simulink model "PID_Tavola1"  (R2018b)
settings: Solver=FixedStepAuto  StartTime=0.0  StopTime=10  FixedStep=0.1  RelTol=1e-3
values from neighbouring files (symbols this model uses):
  cond_init = [x1,x2,x3,x4,x5,x6]'    [main.m]
  Law = [10,4,4,4,4,4 ... (first row only)    [main.m]
  param = param'    [main.m]
settings Model: Creator=AmatoPi  LastModifiedBy=Utente

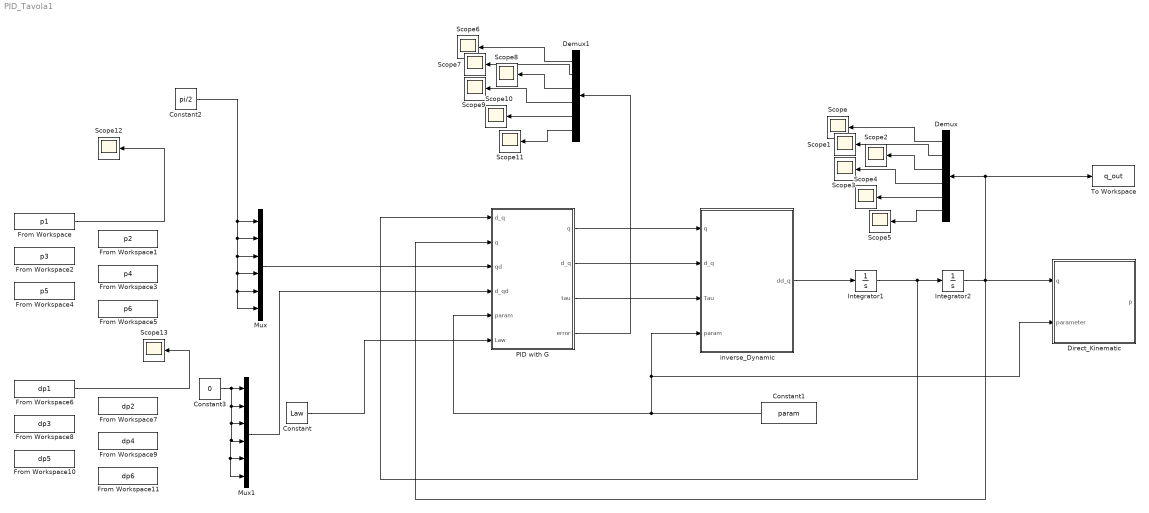
== system PID_Tavola1 ==
  Constant : Constant  Value=Law
  Constant1 : Constant  Value=param
  Constant2 : Constant  Value=pi/2
  Constant3 : Constant  Value=0
  Demux : Demux  Outputs=6
  Demux1 : Demux  Outputs=6
  Direct_Kinematic : MATLAB Function  TreatAsAtomicUnit=on
  From Workspace : FromWorkspace  VariableName=p1  SampleTime=0
  From Workspace1 : FromWorkspace  VariableName=p2  SampleTime=0
  From Workspace10 : FromWorkspace  VariableName=dp5  SampleTime=0
  From Workspace11 : FromWorkspace  VariableName=dp6  SampleTime=0
  From Workspace2 : FromWorkspace  VariableName=p3  SampleTime=0
  From Workspace3 : FromWorkspace  VariableName=p4  SampleTime=0
  From Workspace4 : FromWorkspace  VariableName=p5  SampleTime=0
  From Workspace5 : FromWorkspace  VariableName=p6  SampleTime=0
  From Workspace6 : FromWorkspace  VariableName=dp1  SampleTime=0
  From Workspace7 : FromWorkspace  VariableName=dp2  SampleTime=0
  From Workspace8 : FromWorkspace  VariableName=dp3  SampleTime=0
  From Workspace9 : FromWorkspace  VariableName=dp4  SampleTime=0
  Integrator1 : Integrator  InitialCondition=[0;0;0;0;0;0]
  Integrator2 : Integrator  InitialCondition=cond_init
  Mux : Mux  Inputs=6
  Mux1 : Mux  Inputs=6
  PID with G : MATLAB Function  TreatAsAtomicUnit=on
  Scope{,1..13} (14 alike) : Scope
  To Workspace : ToWorkspace  VariableName=q_out  SaveFormat=Timeseries  SampleTime=-1
  inverse_Dynamic : MATLAB Function  TreatAsAtomicUnit=on
  wires:
  PID with G/3(tau) -> inverse_Dynamic/3(Tau)
  PID with G/2(d_q) -> inverse_Dynamic/2(d_q)
  PID with G/1(q) -> inverse_Dynamic/1(q)
  inverse_Dynamic/1(dd_q) -> Integrator1/1
  Integrator1/1 -> PID with G/1("d_q "), Integrator2/1
  Integrator2/1 -> Direct_Kinematic/1(q), To Workspace/1, Demux/1, PID with G/2("q ")
  Constant/1 -> PID with G/6(Law)
  Constant1/1 -> PID with G/5(param), Direct_Kinematic/2(parameter), inverse_Dynamic/4(param)
  Mux/1 -> PID with G/3(qd)
  From Workspace/1 -> Scope12/1
  Demux/1 -> Scope/1
  Demux/2 -> Scope1/1
  Demux/3 -> Scope2/1
  Demux/4 -> Scope3/1
  Demux/5 -> Scope4/1
  Demux/6 -> Scope5/1
  Demux1/5 -> Scope10/1
  Demux1/6 -> Scope11/1
  Demux1/4 -> Scope9/1
  PID with G/4(error) -> Demux1/1
  Demux1/3 -> Scope8/1
  Demux1/2 -> Scope7/1
  Demux1/1 -> Scope6/1
  From Workspace6/1 -> Scope13/1
  Mux1/1 -> PID with G/4(d_qd)
  Constant2/1 -> Mux/6, Mux/5, Mux/4, Mux/3, Mux/2, Mux/1
  Constant3/1 -> Mux1/6, Mux1/5, Mux1/4, Mux1/3, Mux1/2, Mux1/1

== matlab function PID_Tavola1/PID with G ==
  data: q output; d_q output; d_q input; tau output; q input; qd input; d_qd input; param input; Law input; error output
function [q,d_q,tau,error]  = PID_Contro(d_q, q, qd, d_qd, param, Law)
       
    kp = 8*eye(6);
    kd = 2*eye(6);
    [~,~,G] = Dinamica(param,q,d_q);
    
    error = qd - q;
    d_error = d_qd - d_q;
  
    tau = kp*error + G + kd*d_error ;
    
end

== matlab function PID_Tavola1/inverse_Dynamic ==
  data: q input; dd_q output; d_q input; Tau input; param input
function dd_q = inverseDynamic(q,d_q,Tau,param)
    
    [B,C,G] = Dinamica(param,q,d_q);

    tot = Tau - C*d_q - G;    
    dd_q = B\(tot);

end

== matlab function PID_Tavola1/Direct_Kinematic ==
  data: q input; p output; parameter input
function p = DirectK(q,parameter)

	[p,com,head] = Direct_Kinematics(parameter,q);
    
    

end
